simulink model "HelloWorldNew"  (Simulink 7.4)
settings: Solver=FixedStepDiscrete  StartTime=0.0  StopTime=30  FixedStep=1  MaxStep=1  RelTol=1e-3
undefined symbols (not defined in the file or in its folder): uk, xk
libraries: BLOM_Lib x8
settings Model: Creator=vichik  LastModifiedBy=Kyle
settings OptimizationCC: InitFltsAndDblsToZero=on

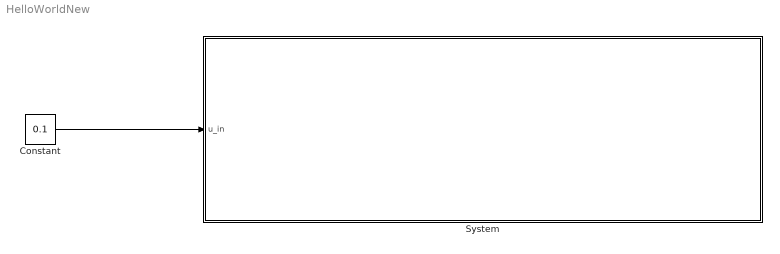
== system HelloWorldNew ==
  Constant : Constant  Value=0.1
  System : Subsystem
  wires:
  Constant/1 -> System/1(u_in)

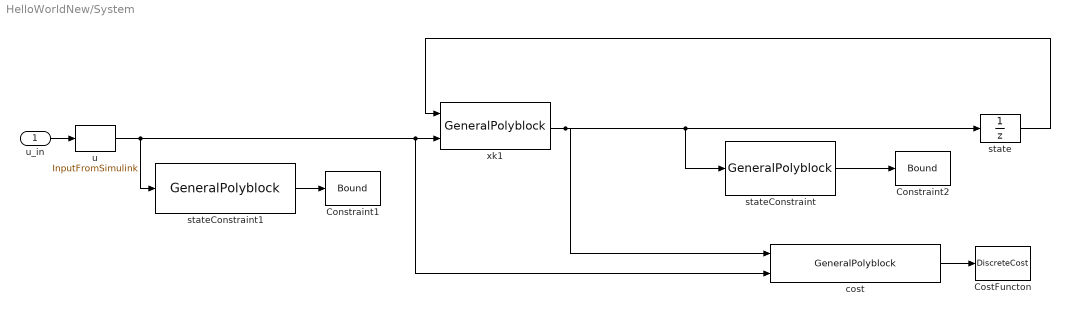
== system HelloWorldNew/System ==
  u_in : Inport
  Constraint1 : BLOM_Lib/Bound  SystemSampleTime=-1  ub=0  lb=-inf  initial_step=on  final_step=on  intermediate_step=on
  Constraint2 : BLOM_Lib/Bound  SystemSampleTime=-1  ub=0  lb=-inf  initial_step=on  final_step=on  intermediate_step=on
  CostFuncton : BLOM_Lib/DiscreteCost  SystemSampleTime=-1  initial_step=on  final_step=on  intermediate_step=on
  cost : BLOM_Lib/GeneralPolyblock  SystemSampleTime=-1  P_f=[2 0; 0 2]  K_f=[0.5 2]  P_g=[0 0 ]  K_g=1  inputs=xk,uk  inputScalar=on  outputScalar=on
  state : UnitDelay  X0=1  SampleTime=-1
  stateConstraint : BLOM_Lib/GeneralPolyblock  SystemSampleTime=-1  P_f="[1  ;  0 ]"  K_f=[1 -1 ; -1 0.5 ]  P_g="[0  ]"  K_g=1  inputs=x  inputScalar=on  outputScalar=off
  stateConstraint1 : BLOM_Lib/GeneralPolyblock  SystemSampleTime=-1  P_f="[1  ;  0 ]"  K_f=[1 -2 ; -1 -2 ]  P_g="[0  ]"  K_g=1  inputs=u  inputScalar=on  outputScalar=off
  u : BLOM_Lib/InputFromSimulink  SystemSampleTime=-1  interpType=Zero-Order Hold
  xk1 : BLOM_Lib/GeneralPolyblock  SystemSampleTime=-1  P_f=[1 0; 0 1]  K_f=[0.9 1]  P_g=[0 0 ]  K_g=[1]  inputs=xk,uk  inputScalar=on  outputScalar=on
  wires:
  xk1/1 -> cost/1, state/1, stateConstraint/1
  state/1 -> xk1/1
  u/1 -> xk1/2, cost/2, stateConstraint1/1
  cost/1 -> CostFuncton/1
  stateConstraint/1 -> Constraint2/1
  u_in/1 -> u/1
  stateConstraint1/1 -> Constraint1/1
